simulink model "BearinglessMotorSimulation"  (R2024b)
settings: Solver=FixedStepAuto  StartTime=0  StopTime=Tend  FixedStep=Tsim  RelTol=1e-3
values from neighbouring files (symbols this model uses):
  fx_cmd = 9    [setup.m]
  fx_end = (2/6)*Tend    (= 0.01)    [setup.m]
  fx_start = 0    [setup.m]
  fy_cmd = 9    [setup.m]
  fy_end = (5/6)*Tend    (= 0.025)    [setup.m]
  fy_start = (3/6)*Tend    (= 0.015)    [setup.m]
  p = 4    [setup.m]    (also in setup_actuator_2026.m = 7; setup_ismb_19.m)
  rotor_unbalance_pos = 0    [setup.m]
  rotor_unbalance_weight = 1    [setup.m]
  speed_cmd = 7500    [setup.m]
  torque_cmd = 0.2    [setup.m]
  torque_end = (4/6)*Tend    (= 0.02)    [setup.m]
  torque_start = (1/6)*Tend    (= 0.005)    [setup.m]
  V_DC = 160    [setup.m]    (also in setup_actuator_2026.m; setup_ismb_19.m)
settings Model: Creator=chiba  LastModifiedBy=mhmok
settings SolverCC: AllowMultiTaskInputOutput=on
settings OptimizationCC: DefaultParameterBehavior=Inlined  ReuseModelBlockBuffer=off  EnhancedBackFolding=on  PassReuseOutputArgsAs=Individual arguments  ZeroExternalMemoryAtStartup=off  ZeroInternalMemoryAtStartup=off  OptimizeBlockOrder=speed  DifferentSizesBufferReuse=on  EfficientTunableParamExpr=on
settings DebuggingCC: ParameterTunabilityLossMsg=error
settings SFSimCC: MATLABDynamicMemAlloc=off
settings RTWCC: Description=Embedded Coder  SystemTargetFile=ert.tlc  TemplateMakefile=ert_default_tmf  GPUComputeCapability=3.5
settings CodeAppCC: ForceParamTrailComments=on  IgnoreCustomStorageClasses=off  OperatorAnnotations=on  SimulinkDataObjDesc=on  SFDataObjDesc=on  InsertBlockDesc=on
settings ERTTargetCC: TargetLangStandard=C99 (ISO)  ERTCustomFileTemplate=example_file_process.tlc  DynamicArrayContainerType=coder::array

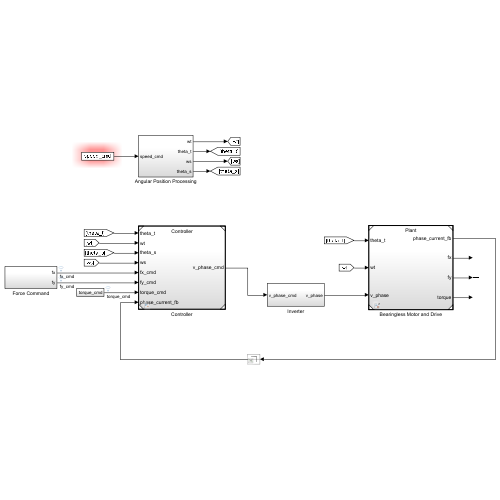
[thumbnail: Simulink's stored preview of the top-level diagram]
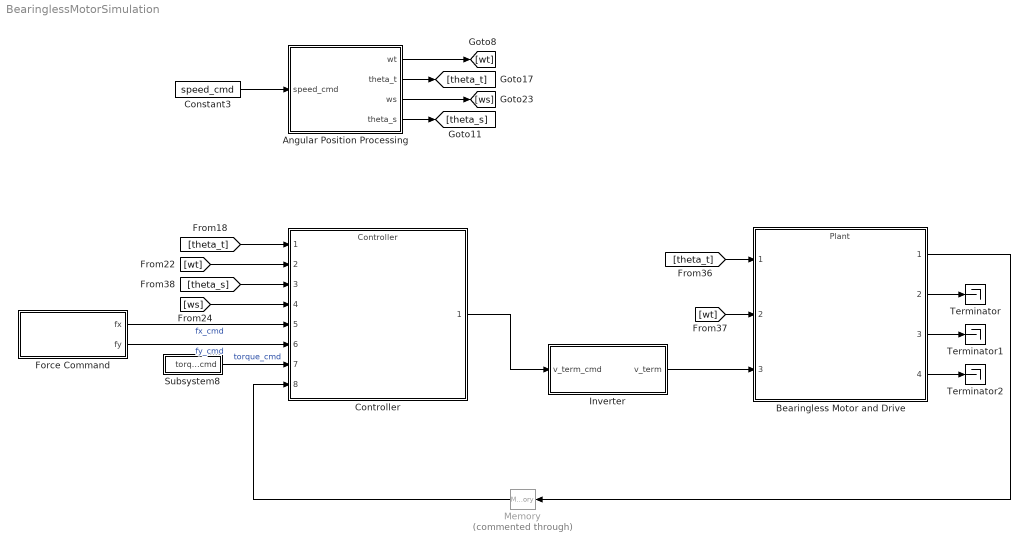
== system BearinglessMotorSimulation ==
  Angular Position Processing : Subsystem
  Bearingless Motor and Drive : ModelReference  ModelNameDialog=Plant  SimulationMode=Normal  ModelReferenceVersion=5.238
  Constant3 : Constant  Value=speed_cmd
  Controller : ModelReference  ModelNameDialog=Controller  SimulationMode=Normal  ModelReferenceVersion=5.271
  Force Command : Subsystem
  Inverter : Subsystem
  Memory : Memory  Commented=through
  Subsystem8 : Subsystem
  Terminator : Terminator
  Terminator1 : Terminator
  Terminator2 : Terminator
  wires:
  Constant3/1 -> Angular Position Processing/1(speed_cmd)
  Angular Position Processing/1(wt) -> [wt]
  Angular Position Processing/2(theta_t) -> [theta_t]
  Angular Position Processing/3(ws) -> [ws]
  Angular Position Processing/4(theta_s) -> [theta_s]
  [wt] -> Bearingless Motor and Drive/2
  [theta_t] -> Bearingless Motor and Drive/1
  [theta_t] -> Controller/1
  [wt] -> Controller/2
  [theta_s] -> Controller/3
  [ws] -> Controller/4
  Subsystem8/1(torque_cmd) -> Controller/7  "torque_cmd"
  Bearingless Motor and Drive/2 -> Terminator/1
  Bearingless Motor and Drive/3 -> Terminator1/1
  Bearingless Motor and Drive/4 -> Terminator2/1
  Bearingless Motor and Drive/1 -> Memory/1
  Memory/1 -> Controller/8
  Force Command/1(fx) -> Controller/5  "fx_cmd"
  Force Command/2(fy) -> Controller/6  "fy_cmd"
  Controller/1 -> Inverter/1(v_term_cmd)
  Inverter/1(v_term) -> Bearingless Motor and Drive/3

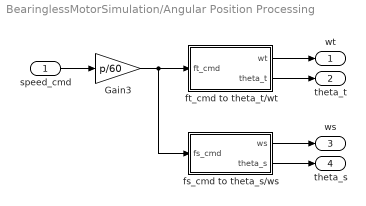
== system BearinglessMotorSimulation/Angular Position Processing ==
  speed_cmd : Inport
  Gain3 : Gain  Gain=p/60
  fs_cmd to theta_s/ws : Subsystem
  ft_cmd to theta_t/wt : Subsystem
  wt : Outport
  theta_t : Outport  Port=2
  ws : Outport  Port=3
  theta_s : Outport  Port=4
  wires:
  ft_cmd to theta_t/wt/1(wt) -> wt/1
  fs_cmd to theta_s/ws/1(ws) -> ws/1
  Gain3/1 -> fs_cmd to theta_s/ws/1(fs_cmd), ft_cmd to theta_t/wt/1(ft_cmd)
  speed_cmd/1 -> Gain3/1
  ft_cmd to theta_t/wt/2(theta_t) -> theta_t/1
  fs_cmd to theta_s/ws/2(theta_s) -> theta_s/1

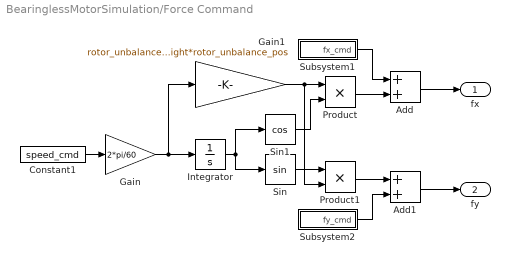
== system BearinglessMotorSimulation/Force Command ==
  Add : Sum
  Add1 : Sum
  Constant1 : Constant  Value=speed_cmd
  Gain : Gain  Gain=2*pi/60
  Gain1 : Gain  Gain=rotor_unbalance_weight*rotor_unbalance_pos
  Integrator : Integrator
  Product : Product
  Product1 : Product
  Sin : Trigonometry
  Sin1 : Trigonometry  Operator=cos
  Subsystem1 : Subsystem
  Subsystem2 : Subsystem
  fx : Outport
  fy : Outport  Port=2
  wires:
  Product1/1 -> Add1/1
  Integrator/1 -> Sin1/1, Sin/1
  Subsystem2/1(fy_cmd) -> Add1/2
  Product/1 -> Add/2
  Gain/1 -> Integrator/1, Gain1/1
  Gain1/1 -> Product1/2, Product/1
  Sin1/1 -> Product/2
  Constant1/1 -> Gain/1
  Add/1 -> fx/1
  Sin/1 -> Product1/1
  Subsystem1/1(fx_cmd) -> Add/1
  Add1/1 -> fy/1

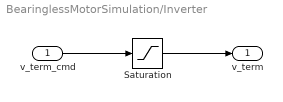
== system BearinglessMotorSimulation/Inverter ==
  v_term_cmd : Inport
  Saturation : Saturate  UpperLimit=V_DC/2  LowerLimit=-V_DC/2
  v_term : Outport
  wires:
  v_term_cmd/1 -> Saturation/1
  Saturation/1 -> v_term/1

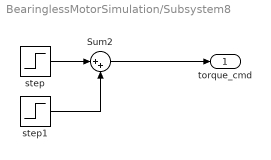
== system BearinglessMotorSimulation/Subsystem8 ==
  Sum2 : Sum  Inputs=|++
  step : Step  Time=torque_start  After=torque_cmd  SampleTime=0
  step1 : Step  Time=torque_end  After=-torque_cmd  SampleTime=0
  torque_cmd : Outport
  wires:
  step1/1 -> Sum2/2
  step/1 -> Sum2/1
  Sum2/1 -> torque_cmd/1

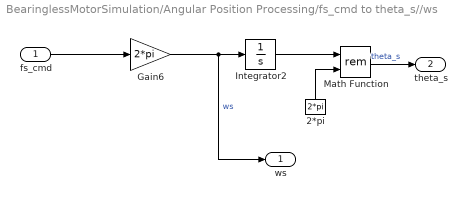
== system BearinglessMotorSimulation/Angular Position Processing/fs_cmd to theta_s//ws ==
  fs_cmd : Inport
  2*pi : Constant  Value=2*pi
  Gain6 : Gain  Gain=2*pi
  Integrator2 : Integrator
  Math Function : Math  Operator=rem  SignedPower=on
  ws : Outport
  theta_s : Outport  Port=2
  wires:
  Gain6/1 -> ws/1, Integrator2/1  "ws"
  2*pi/1 -> Math Function/2
  fs_cmd/1 -> Gain6/1
  Integrator2/1 -> Math Function/1
  Math Function/1 -> theta_s/1  "theta_s"

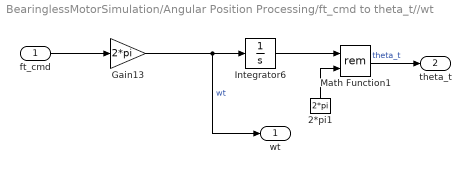
== system BearinglessMotorSimulation/Angular Position Processing/ft_cmd to theta_t//wt ==
  ft_cmd : Inport
  2*pi1 : Constant  Value=2*pi
  Gain13 : Gain  Gain=2*pi
  Integrator6 : Integrator
  Math Function1 : Math  Operator=rem  SignedPower=on
  wt : Outport
  theta_t : Outport  Port=2
  wires:
  Integrator6/1 -> Math Function1/1
  ft_cmd/1 -> Gain13/1
  2*pi1/1 -> Math Function1/2
  Gain13/1 -> wt/1, Integrator6/1  "wt"
  Math Function1/1 -> theta_t/1  "theta_t"

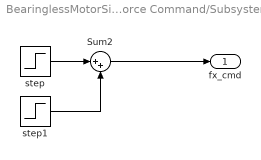
== system BearinglessMotorSimulation/Force Command/Subsystem1 ==
  Sum2 : Sum  Inputs=|++
  step : Step  Time=fx_start  After=fx_cmd  SampleTime=0
  step1 : Step  Time=fx_end  After=-fx_cmd  SampleTime=0
  fx_cmd : Outport
  wires:
  Sum2/1 -> fx_cmd/1
  step/1 -> Sum2/1
  step1/1 -> Sum2/2

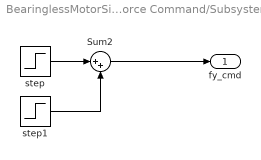
== system BearinglessMotorSimulation/Force Command/Subsystem2 ==
  Sum2 : Sum  Inputs=|++
  step : Step  Time=fy_start  After=fy_cmd  SampleTime=0
  step1 : Step  Time=fy_end  After=-fy_cmd  SampleTime=0
  fy_cmd : Outport
  wires:
  Sum2/1 -> fy_cmd/1
  step/1 -> Sum2/1
  step1/1 -> Sum2/2
